simulink model "BuckBoost1"  (Simulink 8.0)
settings: Solver=FixedStepDiscrete  StartTime=0.0  StopTime=5  FixedStep=1e-5  RelTol=1e-3
values from neighbouring files (symbols this model uses):
  Imax = 16    [BuckBoost1_Init1.m]
  R = 30    [BuckBoost1_Init1.m]
  Ts = 1e-3    (= 0.001)    [BuckBoost1_Init1.m]
  Vin = 40    [BuckBoost1_Init1.m]
libraries: powerlib x12, powerlib_extras x2
settings Model: Creator=zxn  LastModifiedBy=Harri
settings DataIOCC: SignalLoggingSaveFormat=ModelDataLogs
settings DebuggingCC: FcnCallInpInsideContextMsg=UseLocalSettings
settings GRTTargetCC: CombineOutputUpdateFcns=off  GRTInterface=on

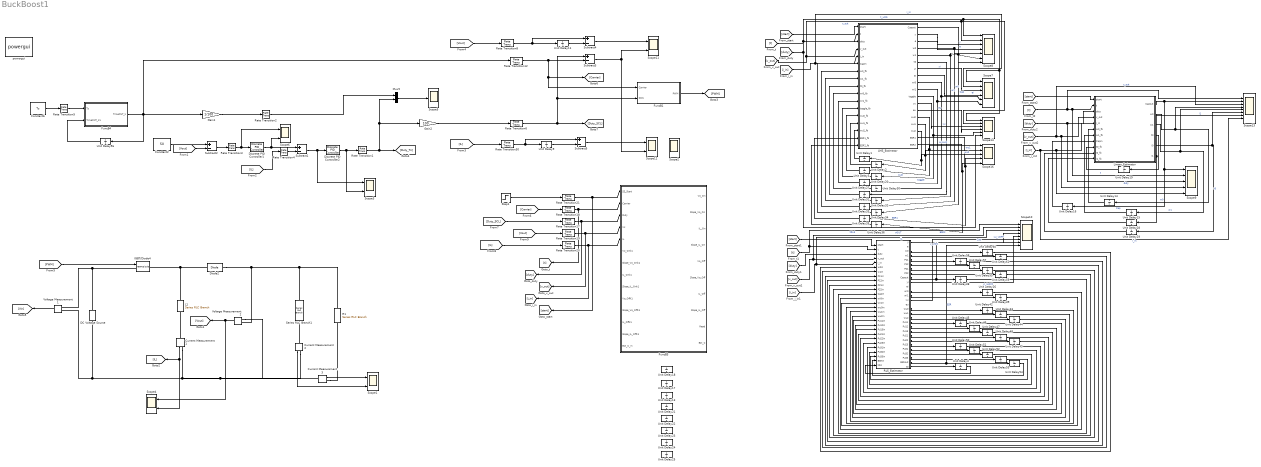
== system BuckBoost1 ==
  Constant2 : Constant  Value=50
  Constant6 : Constant  Value=Ts
  Current Measurement1 : powerlib/Measurements/Current Measurement  PhasorSimulation=off  OutputType=Complex  PSBequivalent=0
  Current Measurement2 : powerlib/Measurements/Current Measurement  PhasorSimulation=off  OutputType=Complex  PSBequivalent=0
  Current Measurement3 : powerlib/Measurements/Current Measurement  PhasorSimulation=off  OutputType=Complex  PSBequivalent=0
  DC Voltage Source : powerlib/Electrical Sources/DC Voltage Source  Amplitude=Vin  Measurements=None
  Diode2 : powerlib/Power Electronics/Diode  Ron=0.001  Lon=0  Vf=0.8  IC=0  UseSnubber=off  Rs=inf  Cs=inf  Measurements=off
  Discrete PID Controller1 : powerlib_extras/Discrete  Control Blocks/Discrete PID Controller  Kp=1.4  Ki=0.4  Kd=0  TcD=0  Par_Limits=[1 -1]*Imax  Init=0  Ts=Ts
  Discrete PID Controller2 : powerlib_extras/Discrete  Control Blocks/Discrete PID Controller  Kp=30e-3  Ki=50e-3  Kd=0  TcD=0  Par_Limits=[1 -1]*0.9  Init=0  Ts=Ts
  FuncB1 : MATLAB Function  TreatAsAtomicUnit=on
  FuncB3 : MATLAB Function  TreatAsAtomicUnit=on
  FuncB4 : MATLAB Function  TreatAsAtomicUnit=on
  Gain1 : Gain  Gain=1/100
  Gain2 : Gain  Gain=100
  IGBT/Diode4 : powerlib/Power Electronics/IGBT//Diode  Ron=1e-3  Rs=1e5  Cs=inf  Measurements=off
  L1 : powerlib/Elements/Series RLC Branch  LConnTagsString=__new0  RConnTagsString=__new0  BranchType=L  Resistance=1  Inductance=5e-3  SetiL0=off  InitialCurrent=0  Capacitance=1e-6  Setx0=off  InitialVoltage=0  Measurements=None
  LMS_Estimator : MATLAB Function  TreatAsAtomicUnit=on
  Linear_Estimator : MATLAB Function  TreatAsAtomicUnit=on
  Mux5 : Mux  Inputs=2
  R1 : powerlib/Elements/Series RLC Branch  LConnTagsString=__new0  RConnTagsString=__new0  BranchType=R  Resistance=R  Inductance=1e-3  SetiL0=off  InitialCurrent=0  Capacitance=1e-6  Setx0=off  InitialVoltage=0  Measurements=None
  RLS_Estimator : MATLAB Function  TreatAsAtomicUnit=on
  Rate Transition{1..2,6,8,12,17..21,30} (11 alike) : RateTransition  OutPortSampleTime=1e-5
  Rate Transition3 : RateTransition  OutPortSampleTime=Ts
  Rate Transition4 : RateTransition  OutPortSampleTime=Ts
  Rate Transition5 : RateTransition  X0=Ts  OutPortSampleTime=1e-5
  Scope{1,3..4,6,11..12} (6 alike) : Scope  NumInputPorts=2
      Scope1 settings: TickLabels=on  TimeRange=10  YMin=210~0  YMax=320~47.5  SaveName=var1
      Scope11 settings: TickLabels=on  TimeRange=5  YMin=-0.06~-40  YMax=0.07~65  SaveName=var10  MaxDataPoints=1000000
      Scope12 settings: TickLabels=on  TimeRange=5  YMin=-0.011~-40  YMax=0.01~65  SaveName=var13  MaxDataPoints=1000000
      Scope3 settings: TickLabels=on  TimeRange=1.5  YMin=0.5~0  YMax=0.605~1  SaveName=var4
      Scope4 settings: TickLabels=on  YMin=0~-1  YMax=52.5~12  SaveName=var
      Scope6 settings: TickLabels=on  TimeRange=1.5  YMin=0.5~0  YMax=0.605~1  SaveName=var2
  Scope10 : Scope  NumInputPorts=8
      settings: TickLabels=on  TimeRange=5  YMin=0~0~0~49.7~0~-5~-5~-5  YMax=100~0.0015~55~50.1~75~5~5~5  SaveName=var9  MaxDataPoints=1000000
  Scope13 : Scope  NumInputPorts=8
      settings: TickLabels=on  TimeRange=5  YMin=0~-1~49.7~49.7~-5~-5~-5~-5  YMax=100~-0.4~50.1~50.1~5~5~5~5  SaveName=var8  MaxDataPoints=1000000
  Scope14 : Scope  NumInputPorts=6
      settings: TickLabels=on  TimeRange=2  YMin=0~-1~49.7~49.7~-1~-5  YMax=100~-0.4~50.1~50.1~2~5  SaveName=var12  MaxDataPoints=1000000
  Scope16 : Scope  NumInputPorts=5
      settings: TickLabels=on  TimeRange=5  YMin=0~-1~49.7~49.7~-5  YMax=100~-0.4~50.1~50.1~5  SaveName=var15  MaxDataPoints=1000000
  Scope2 : Scope  NumInputPorts=4
      settings: TickLabels=on  TimeRange=5  YMin=-0.011~-40~-5~-5  YMax=0.01~65~5~5  SaveName=var3  MaxDataPoints=1000000
  Scope5 : Scope
      settings: TickLabels=on  TimeRange=1.5  YMin=0.5  YMax=0.605  SaveName=var5  MaxDataPoints=100000
  Scope7 : Scope  NumInputPorts=6
      settings: TickLabels=on  TimeRange=5  YMin=0~-1~49.7~49.7~-0.1~-5  YMax=100~-0.4~50.1~50.1~0.1~5  SaveName=var6  MaxDataPoints=1000000
  Scope8 : Scope  NumInputPorts=7
      settings: TickLabels=on  TimeRange=5  YMin=0~-1~49.7~49.7~-0.1~-5~-5  YMax=100~-0.4~50.1~50.1~0.1~5~5  SaveName=var7  MaxDataPoints=1000000
  Scope9 : Scope  NumInputPorts=5
      settings: TickLabels=on  TimeRange=5  YMin=0~-10~-10~0~0  YMax=5~110~110~100~10  SaveName=var11  MaxDataPoints=1000000
  Series RLC Branch1 : powerlib/Elements/Series RLC Branch  LConnTagsString=__new0  RConnTagsString=__new0  BranchType=RC  Resistance=75e-3*1  Inductance=1e-3  SetiL0=off  InitialCurrent=0  Capacitance=1e-3*1.25  Setx0=off  InitialVoltage=500  Measurements=None
  Step1 : Step  Time=3.3  SampleTime=0
  Subtract1 : Sum  Inputs=+-  SampleTime=Ts
  Subtract{2..5} (4 alike) : Sum  Inputs=+-
  Unit Delay{1..4,9,11,13..36,38..39,42..44,46..48,50..52,54..57,60..61} (47 alike) : UnitDelay  SampleTime=1e-5
  Unit Delay{45,49,53,58..59} (5 alike) : UnitDelay  InitialCondition=100  SampleTime=1e-5
  Voltage Measurement1 : powerlib/Measurements/Voltage Measurement  PhasorSimulation=off  OutputType=Complex  PSBequivalent=0
  Voltage Measurement2 : powerlib/Measurements/Voltage Measurement  PhasorSimulation=off  OutputType=Complex  PSBequivalent=0
  powergui : powerlib/powergui  Priority=2  SimulationMode=Discrete  SolverType=Tustin  SampleTime=1e-5  frequency=60  SPID=off  DisableSnubberDevices=off  DisableRonSwitches=off  DisableVfSwitches=off  SwTol=0  Interpol=off  DisplayEquations=off  FunctionMessages=off  frequencyindice=0  Pbase=100e6  ErrMax=1e-4  Iterations=50  UnitsV=kV  UnitsW=MW  echomessages=off  HookPort=off  EnableUseOfTLC=off  x0status=blocks  RestoreLinks=warning  ResistiveCurrentMeasurement=off  Frange=[0:2:500]  Ylog=off  Xlog=off  ShowGrid=off  save=off  variable=ZData  structure=ScopeData  ZoomFFT=on  StartTime=0.0  cycles=1  DisplayStyle=1  fundamental=60  FreqAxis=off  MaxFrequency=8000  frequencyindicesteady=1  RmsSteady=1  display=off  Ts=0  methode=off
  wires:
  Constant2/1 -> Subtract2/1
  Subtract2/1 -> Rate Transition3/1
  Voltage Measurement2/1 -> Scope4/1, [Vout]
  Current Measurement1/1 -> [IL], Scope4/2
  Current Measurement3/1 -> Scope1/1
  Current Measurement2/1 -> Scope1/2
  Rate Transition2/1 -> Mux5/1
  Rate Transition3/1 -> Discrete PID Controller1/1, Scope6/1
  Discrete PID Controller1/1 -> Subtract1/1, Scope6/2
  Subtract1/1 -> Discrete PID Controller2/1, Scope3/1
  Rate Transition4/1 -> Subtract1/2
  [IL] -> Rate Transition4/1
  [Vout] -> Subtract2/2
  Discrete PID Controller2/1 -> Rate Transition1/1, Scope3/2
  Rate Transition1/1 -> Mux5/2, Gain2/1, [Duty_Ts]
  Mux5/1 -> Scope5/1
  Rate Transition6/1 -> [Duty_SCL], Subtract3/1, FuncB1/2(Duty)
  Rate Transition8/1 -> Unit Delay11/1, Subtract4/1
  [PWM] -> IGBT/Diode4/1
  Voltage Measurement1/1 -> [Vin]
  Rate Transition5/1 -> FuncB4/1(Ts)
  Constant6/1 -> Rate Transition5/1
  Unit Delay56/1 -> FuncB4/2(TimeCNT_k1)
  FuncB4/1(TimeCNT_k) -> Unit Delay56/1, Gain1/1, Rate Transition12/1
  Gain1/1 -> Rate Transition2/1
  Gain2/1 -> Rate Transition6/1
  Subtract3/1 -> Scope11/2, Scope12/2
  Rate Transition12/1 -> Subtract3/2, [Carrier], FuncB1/1(Carrier)
  Unit Delay11/1 -> Subtract4/2
  Subtract4/1 -> Scope11/1
  [Vout] -> Rate Transition8/1
  [Carrier] -> Rate Transition18/1
  [Duty_SCL] -> Rate Transition17/1
  Step1/1 -> Rate Transition21/1
  [IL] -> Rate Transition20/1
  [Vout] -> Rate Transition19/1
  FuncB1/1(PWM) -> [PWM]
  Rate Transition21/1 -> [start], FuncB3/1(SS_Start)
  Rate Transition19/1 -> [v_out], FuncB3/4(Vc)
  Rate Transition20/1 -> [i_in], FuncB3/5(IL)
  [IL] -> Rate Transition30/1
  Unit Delay9/1 -> Subtract5/2
  Rate Transition30/1 -> Unit Delay9/1, Subtract5/1
  Subtract5/1 -> Scope12/1
  Rate Transition17/1 -> [duty], FuncB3/3(Duty)
  Rate Transition18/1 -> [t], FuncB3/2(Carrier)
  [start] -> RLS_Estimator/1(start)
  [t] -> RLS_Estimator/2(t), Scope10/1  "tRLS"
  [duty] -> RLS_Estimator/3(duty)
  [v_out] -> Scope10/2, RLS_Estimator/4(v_out)  "vOUT"
  [i_in] -> Scope10/3, RLS_Estimator/5(i_in)  "iL"
  [i_in] -> Scope13/8, Scope9/5, Linear_Estimator/5(i_in)  "i_in"
  [v_out] -> Scope13/3, Scope9/4, Linear_Estimator/4(v_out)  "v_out"
  [duty] -> Scope9/3, Linear_Estimator/3(duty)  "duty"
  [t] -> Scope13/1, Scope9/2, Linear_Estimator/2(t)  "t"
  Linear_Estimator/1(Capout) -> Scope13/2, Unit Delay16/1, Scope9/1  "Cap"
  [start] -> Linear_Estimator/1(start)
  Unit Delay14/1 -> Linear_Estimator/6(w0_fb)
  Unit Delay15/1 -> Linear_Estimator/7(w1_fb)
  Unit Delay16/1 -> Linear_Estimator/8(Capin)
  Linear_Estimator/3(w1) -> Scope13/5, Unit Delay15/1  "w1"
  Linear_Estimator/2(w0) -> Scope13/4, Unit Delay14/1  "w0"
  Linear_Estimator/4(t0) -> Unit Delay19/1
  Unit Delay19/1 -> Linear_Estimator/9(t0_fb)
  Linear_Estimator/6(i1) -> Unit Delay28/1, Scope13/7  "i1"
  Unit Delay28/1 -> Linear_Estimator/11(i1_fb)
  Linear_Estimator/5(i0) -> Scope13/6, Unit Delay29/1  "i0"
  Unit Delay29/1 -> Linear_Estimator/10(i0_fb)
  LMS_Estimator/16(wu2) -> Scope16/3, Unit Delay1/1  "wu2"
  Unit Delay1/1 -> LMS_Estimator/15(wu2_fb)
  LMS_Estimator/15(wu1) -> Unit Delay2/1, Scope16/2  "wu1"
  Unit Delay2/1 -> LMS_Estimator/14(wu1_fb)
  LMS_Estimator/14(wu0) -> Scope16/1, Unit Delay3/1  "wu0"
  Unit Delay3/1 -> LMS_Estimator/13(wu0_fb)
  LMS_Estimator/11(toggle) -> Scope14/5, Unit Delay20/1  "toggle"
  Unit Delay20/1 -> LMS_Estimator/12(toggle_fb)
  LMS_Estimator/10(wi1) -> Scope7/6, Unit Delay27/1  "wi1"
  Unit Delay27/1 -> LMS_Estimator/11(wi1_fb)
  LMS_Estimator/9(wi0) -> Scope7/5, Unit Delay30/1  "wi0"
  Unit Delay30/1 -> LMS_Estimator/10(wi0_fb)
  LMS_Estimator/6(t0) -> Unit Delay31/1
  Unit Delay31/1 -> LMS_Estimator/9(t0_fb)
  LMS_Estimator/5(w1) -> Unit Delay32/1, Scope8/6  "w1"
  Unit Delay32/1 -> LMS_Estimator/8(w1_fb)
  LMS_Estimator/4(w0) -> Scope8/5, Unit Delay33/1  "w0"
  Unit Delay33/1 -> LMS_Estimator/7(w0_fb)
  LMS_Estimator/1(Capout) -> Scope8/7, Unit Delay34/1  "Cap"
  Unit Delay34/1 -> LMS_Estimator/6(Capin)
  [start] -> LMS_Estimator/1(start)
  [t] -> Scope8/1, Scope14/1, Scope7/1, LMS_Estimator/2(t)  "t_LMS"
  [duty] -> Scope14/6, LMS_Estimator/3(duty)
  [v_out] -> Scope14/2, Scope8/2, LMS_Estimator/4(v_out)  "v_out"
  [i_in] -> LMS_Estimator/5(i_in), Scope7/2  "i_in"
  LMS_Estimator/2(y) -> Scope8/3  "y"
  LMS_Estimator/3(e) -> Scope8/4  "e"
  LMS_Estimator/7(yi) -> Scope7/3  "yi"
  LMS_Estimator/8(ei) -> Scope7/4  "ei"
  LMS_Estimator/12(yu) -> Scope14/3  "yu"
  LMS_Estimator/13(eu) -> Scope14/4  "eu"
  LMS_Estimator/17(ESR1) -> Unit Delay35/1, Scope16/4  "ESR1"
  LMS_Estimator/18(ESR2) -> Unit Delay36/1, Scope16/5  "ESR2"
  Unit Delay35/1 -> LMS_Estimator/16(ESR1_fb)
  Unit Delay36/1 -> LMS_Estimator/17(ESR2_fb)
  RLS_Estimator/3(w0) -> Unit Delay60/1
  RLS_Estimator/4(w1) -> Unit Delay61/1
  RLS_Estimator/5(P11) -> Unit Delay58/1
  RLS_Estimator/6(P12) -> Unit Delay57/1
  RLS_Estimator/7(P21) -> Unit Delay55/1
  RLS_Estimator/8(P22) -> Unit Delay59/1
  RLS_Estimator/28(ESRout) -> Scope10/8, Unit Delay54/1  "ESR"
  RLS_Estimator/27(Pu33) -> Unit Delay53/1
  RLS_Estimator/26(Pu32) -> Unit Delay52/1
  RLS_Estimator/25(Pu31) -> Unit Delay51/1
  RLS_Estimator/24(Pu23) -> Unit Delay50/1
  RLS_Estimator/23(Pu22) -> Unit Delay49/1
  RLS_Estimator/22(Pu21) -> Unit Delay48/1
  RLS_Estimator/21(Pu13) -> Unit Delay47/1
  RLS_Estimator/20(Pu12) -> Unit Delay46/1
  RLS_Estimator/19(Pu11) -> Unit Delay45/1
  RLS_Estimator/18(wu2) -> Unit Delay44/1
  RLS_Estimator/17(wu1) -> Unit Delay43/1
  RLS_Estimator/16(wu0) -> Unit Delay42/1
  RLS_Estimator/13(wi1) -> Unit Delay39/1
  RLS_Estimator/12(wi0) -> Unit Delay26/1
  RLS_Estimator/9(Capout) -> Scope10/7, Unit Delay38/1  "Cap"
  Unit Delay54/1 -> RLS_Estimator/27(ESRin)
  Unit Delay53/1 -> RLS_Estimator/26(Pu33in)
  Unit Delay52/1 -> RLS_Estimator/25(Pu32in)
  Unit Delay51/1 -> RLS_Estimator/24(Pu31in)
  Unit Delay50/1 -> RLS_Estimator/23(Pu23in)
  Unit Delay49/1 -> RLS_Estimator/22(Pu22in)
  Unit Delay48/1 -> RLS_Estimator/21(Pu21in)
  Unit Delay47/1 -> RLS_Estimator/20(Pu13in)
  Unit Delay46/1 -> RLS_Estimator/19(Pu12in)
  Unit Delay45/1 -> RLS_Estimator/18(Pu11in)
  Unit Delay44/1 -> RLS_Estimator/17(wu2in)
  Unit Delay43/1 -> RLS_Estimator/16(wu1in)
  Unit Delay42/1 -> RLS_Estimator/15(wu0in)
  Unit Delay39/1 -> RLS_Estimator/14(wi1in)
  Unit Delay26/1 -> RLS_Estimator/13(wi0in)
  Unit Delay38/1 -> RLS_Estimator/12(Capin)
  Unit Delay59/1 -> RLS_Estimator/11(P22in)
  Unit Delay55/1 -> RLS_Estimator/10(P21in)
  Unit Delay57/1 -> RLS_Estimator/9(P12in)
  Unit Delay58/1 -> RLS_Estimator/8(P11in)
  Unit Delay61/1 -> RLS_Estimator/7(w1in)
  Unit Delay60/1 -> RLS_Estimator/6(w0in)
  RLS_Estimator/1(y) -> Scope10/4  "y_vON"
  RLS_Estimator/10(yi) -> Scope10/5  "yi_iLOFF"
  RLS_Estimator/14(yu) -> Scope10/6  "yu_vOFF"
  RLS_Estimator/29(t0) -> Unit Delay4/1
  Unit Delay4/1 -> RLS_Estimator/28(t0in)
  connections:
  DC Voltage Source/RConn1 -- IGBT/Diode4/LConn1 -- Voltage Measurement1/LConn1
  Diode2/RConn1 -- IGBT/Diode4/RConn1 -- L1/RConn1
  Current Measurement3/LConn1 -- Current Measurement2/RConn1 -- Voltage Measurement2/LConn1 -- Current Measurement1/RConn1 -- DC Voltage Source/LConn1 -- Voltage Measurement1/LConn2
  Current Measurement1/LConn1 -- L1/LConn1
  Diode2/LConn1 -- R1/RConn1 -- Series RLC Branch1/RConn1 -- Voltage Measurement2/LConn2
  Current Measurement2/LConn1 -- Series RLC Branch1/LConn1
  Current Measurement3/RConn1 -- R1/LConn1

== matlab function LMS_Estimator ==
  data: start input double; t input double; duty input double; Capout output double; y output double; e output double; v_out input double; i_in input double; Capin input double; w0_fb input double; w1_fb input double; w0 output double; w1 output double; t0_fb input double; t0 output double; yi output double; ei output double; wi0_fb input double; wi1_fb input double; wi0 output double; wi1 output double; toggle_fb input double; wu0_fb input double; wu1_fb input double; wu2_fb input double; toggle output double; yu output double; eu output double; wu0 output double; wu1 output double; wu2 output double; ESR1 output double; ESR2 output double; ESR1_fb input double; ESR2_fb input double
function [Capout, y, e, w0, w1, t0, yi, ei, wi0, wi1, toggle, yu, eu, wu0, wu1, wu2, ESR1, ESR2]  = Est_LMS(start,t,duty,v_out,i_in, Capin, w0_fb, w1_fb, t0_fb, wi0_fb, wi1_fb, toggle_fb, wu0_fb, wu1_fb, wu2_fb, ESR1_fb, ESR2_fb)
%#codegen

% LMS parameter
beta = 0.5;
%(good, let see other value)0.1;
%(good, but w1 still oscilating)0.01;
%(better-but-wrong)0.001;%0.0000001;

% timing control
offset = t - duty;

OFFSET_ON_START_abs = 0+5; % for t
OFFSET_ON_END_rel = -5; % for offset
OFFSET_OFF_START_rel = 5; % for offset
OFFSET_OFF_END_abs = 90+5; % for t


% estimate uoON(t) = w0 + w1*t
y = 0.0;
e = 0.0;
w = transpose(zeros(1,2));
w(1) = w0_fb;
w(2) = w1_fb;
w0 = w0_fb;
w1 = w1_fb;

% estimate iLOFF(t) = wi0 + wi1*t
yi = 0.0;
ei = 0.0;

wi = transpose(zeros(1,2));
wi(1) = wi0_fb;
wi(2) = wi1_fb;
wi0 = wi0_fb;
wi1 = wi1_fb;

% estimate uoOFF(t) = wu0 + wu1*t + wu2*t^2
yu = 0.0;
eu = 0.0;

wu = transpose(zeros(1,3));
wu(1) = wu0_fb;
wu(2) = wu1_fb;
wu(3) = wu2_fb;
wu0 = wu0_fb;
wu1 = wu1_fb;
wu2 = wu2_fb;

% ---

% input for uoON(t) and iLOFF(t), i.e. first-order
x = transpose(zeros(1,2));
x(1) = 1;
x(2) = t;
% input for uoOFF(t), i.e. second-order
u = transpose(zeros(1,3));
u(1) = 1;
u(2) = t;
u(3) = t*t;

% some storage...
t0 = t0_fb;
toggle = toggle_fb;
Capout = Capin; %0; % to avoid error on "unconnected path... something..."

% misc
ESR1 = ESR1_fb;
ESR2 = ESR2_fb;

if(start==1)
    if(toggle == 0)
        % FIRST cycle
        
        if(t > OFFSET_ON_START_abs && offset < OFFSET_ON_END_rel) % ON
            % estimate the "C"
            if (t <= OFFSET_ON_START_abs+2) % give some margin
                t0 = t;
            end
            % --- start of LMS_for_uON(t) ---
            % IMPORTANT: offsetting to zero give good estimation result!
            x(2) = t - t0;

            rms = (x(1)^2+x(2)^2)/2;
            y = w'*x;

            e = v_out - y;

            w = w + beta*e*x/rms;
            w0 = w(1);
            w1 = w(2);
            % --- end of LMS_for_uON(t) ---

        elseif(offset >= OFFSET_ON_END_rel && offset <= OFFSET_ON_END_rel+1)
            Capout = -w0/w1/30*10^(-6) * 1000;%R=30
        end
        if(offset > OFFSET_OFF_START_rel && t < OFFSET_OFF_END_abs) % OFF
            % estimate the "ESR"
            if (offset <= OFFSET_OFF_START_rel+2)
                t0 = t;
            end

            % --- start of LMS_for_iL(t) ---
            x(2) = t - t0;

            rms = (x(1)^2+x(2)^2)/2;
            yi = wi'*x;

            ei = i_in - yi;

            wi = wi + beta*ei*x/rms;
            wi0 = wi(1);
            wi1 = wi(2);
            % --- end of LMS_for_iL(t)---
        %elseif(t >= OFFSET_OFF_END_abs && t <= OFFSET_OFF_END_abs+2)
        %    toggle = 1;
        end
        
        if(t >= OFFSET_OFF_END_abs && t <= OFFSET_OFF_END_abs+2)
            toggle = 1;
        end
        
    elseif(toggle == 1)
        % SECOND cycle
        
        if(offset > OFFSET_OFF_START_rel && t < OFFSET_OFF_END_abs) % OFF
            % estimate the u0(t) in OFF condition
            if (offset <= OFFSET_OFF_START_rel+2)
                t0 = t;
            end

            % --- start of LMS_for_uoOFF(t) ---
            u(2) = t - t0;
            u(3) = (t - t0)*(t - t0);

            rms = (u(1)^2+u(2)^2+u(3)^2)/3;
            yu = wu'*u;

            eu = v_out - yu;

            wu = wu + beta*eu*u/rms;
            wu0 = wu(1);
            wu1 = wu(2);
            wu2 = wu(3);
            % --- end of LMS_for_uoOFF(t)---
        elseif(t >= OFFSET_OFF_END_abs && t <= OFFSET_OFF_END_abs+1)
            %toggle = 0;
            
            R = 30;
            C = Capin;
            a = (2*wu2_fb - wi1_fb*R) / (-wu1_fb - wi1_fb*R*R*C + wi0_fb*R*C*C);
            ESR1 = 1/(a*C) - R;
            
            b = a*wu1_fb + 2*wu2_fb;
            ESR2 = (wi0_fb*C - b) / ((b/R) - wi1_fb);
        end
        
        if(t >= OFFSET_OFF_END_abs && t <= OFFSET_OFF_END_abs+2)
            toggle = 0;
        end
    end
end

== matlab function FuncB3 ==
  data: SS_Start input double; Carrier input double; Duty input double; Vc input double; IL input double; Vo_Onk1 input double; Slope_Vo_Onk1 input double; IL_Onk1 input double; Slope_IL_Onk1 input double; Vo_Offk1 input double; Slope_Vo_Offk1 input double; IL_Offk1 input double; Vo_On output double; Slope_Vo_On output double; IL_On output double; Slope_IL_On output double; Vo_Off output double; Slope_Vo_Off output double; IL_Off output double; Slope_IL_Off output double; Read output double; Slope_IL_Offk1 input double; Est_C output double; Est_C_in input double
function [Vo_On,Slope_Vo_On,IL_On,Slope_IL_On,Vo_Off,Slope_Vo_Off,IL_Off,Slope_IL_Off,Read, Est_C] = Sample(SS_Start,Carrier,Duty,Vc,IL,Vo_Onk1,Slope_Vo_Onk1,IL_Onk1,Slope_IL_Onk1,Vo_Offk1,Slope_Vo_Offk1,IL_Offk1,Slope_IL_Offk1, Est_C_in)

Err1=(Carrier - Duty);  Tsimulation=1e-6;
%DtT_On=Duty*Tsimulation;    DtT_Off=(100 - Duty)*Tsimulation;%%!! 100 should be repaced Correspondingly by CNT_Max
Fix10us=10e-6;
Est_C=Est_C_in;
%Test_Out=Test_Out_in;
if(SS_Start==1)
    if(Err1>=-12)&&(Err1<-11) %%Just After Switch-On; (Err1>=-2)&&(Err1<-1); (Carrier==3)
        Vo_On=Vc; IL_On=IL;
        Read=0;
        Slope_Vo_On=Slope_Vo_Onk1; Slope_IL_On=Slope_IL_Onk1;
        Slope_Vo_Off=Slope_Vo_Offk1; Slope_IL_Off=Slope_IL_Offk1;
        Vo_Off=Vo_Offk1; IL_Off=IL_Offk1;
        Est_C=1;
    elseif((Err1>=-2)&&(Err1<-1)) %%Next moment Switch-Off
        %Slope_Vo_On=(Vc - Vo_Onk1)/DtT_On; Slope_IL_On=(IL - IL_Onk1)/DtT_On;
        Slope_Vo_On=(Vc - Vo_Onk1)/Fix10us; Slope_IL_On=(IL - IL_Onk1)/Fix10us;
        Vo_On=Vo_Onk1; IL_On=IL_Onk1;
        Slope_Vo_Off=Slope_Vo_Offk1; Slope_IL_Off=Slope_IL_Offk1; Read=0; 
        Vo_Off=Vo_Offk1; IL_Off=IL_Offk1;
        Est_C=2;
    elseif(Carrier==89) %%Just After Switch Off; Carrier==98; (Err1>3)&&(Err1<=4)
        Vo_Off=Vc;  IL_Off=IL;
        Slope_Vo_Off=Slope_Vo_Offk1;  Slope_IL_Off=Slope_IL_Offk1;
        Slope_Vo_On=Slope_Vo_Onk1;  Slope_IL_On=Slope_IL_Onk1; Read=0;
        Vo_On=Vo_Onk1; IL_On=IL_Onk1;
    elseif(Carrier==99) %%Next moment Switch-On
        %Slope_Vo_Off=(Vc - Vo_Offk1)/DtT_Off;  Slope_IL_Off=(IL - IL_Offk1)/DtT_Off;
        Slope_Vo_Off=(Vc - Vo_Offk1)/Fix10us;  Slope_IL_Off=(IL - IL_Offk1)/Fix10us;
        Vo_Off=Vo_Offk1;  IL_Off=IL_Offk1;
        Read=1;
        Slope_Vo_On=Slope_Vo_Onk1; Slope_IL_On=Slope_IL_Onk1;
        Vo_On=Vo_Onk1; IL_On=IL_Onk1;
    %elseif(Est_C==1)
    %    Test_Out = 2;
    %elseif(Est_C==2)
    %    Test_Out = 3;
    else
        Vo_On=Vo_Onk1; Slope_Vo_On=Slope_Vo_Onk1; IL_On=IL_Onk1; Slope_IL_On=Slope_IL_Onk1; %%On_Readk1
        Vo_Off=Vo_Offk1;  Slope_Vo_Off=Slope_Vo_Offk1;  IL_Off=IL_Offk1;  Slope_IL_Off=Slope_IL_Offk1; Read=0; %%Off_Readk1
    end
else
    Vo_On=49;  Slope_Vo_On=0.5;  IL_On=4;  Slope_IL_On=0.2;
    Vo_Off=50;  Slope_Vo_Off=0.5;  IL_Off=3.8;  Slope_IL_Off=0.2; Read=0;
end

end

== matlab function RLS_Estimator ==
  data: y output double; e output double; w0 output double; w1 output double; P11 output double; P12 output double; P21 output double; P22 output double; Capout output double; start input double; t input double; duty input double; v_out input double; i_in input double; w0in input double; w1in input double; P11in input double; P12in input double; P21in input double; P22in input double; Capin input double; wi0in input double; wi1in input double; wu0in input double; wu1in input double; wu2in input double; Pu11in input double; Pu12in input double; Pu13in input double; Pu21in input double; Pu22in input double; Pu23in input double; Pu31in input double; Pu32in input double; Pu33in input double; ESRin input double; yi output double; ei output double; wi0 output double; wi1 output double; yu output double; eu output double; wu0 output double; wu1 output double; wu2 output double; Pu11 output double; Pu12 output double; Pu13 output double; Pu21 output double; Pu22 output double; Pu23 output double; Pu31 output double; Pu32 output double; Pu33 output double; ESRout output double; t0in input double; t0 output double
function [y, e, w0, w1, P11, P12, P21, P22, Capout, yi, ei, wi0, wi1, yu, eu, wu0, wu1, wu2, Pu11, Pu12, Pu13, Pu21, Pu22, Pu23, Pu31, Pu32, Pu33, ESRout, t0]  = Est_RLS(start,t,duty,v_out,i_in, w0in, w1in, P11in, P12in, P21in, P22in, Capin, wi0in, wi1in, wu0in, wu1in, wu2in, Pu11in, Pu12in, Pu13in, Pu21in, Pu22in, Pu23in, Pu31in, Pu32in, Pu33in, ESRin, t0in)
%#codegen

% --- Time Partition ---
sampling_time = 1e-5;% 1e-6;

offset = t - duty;

OFFSET_ON_START_abs = 0+5; % for t
OFFSET_ON_END_rel = -5; % for offset
OFFSET_OFF_START_rel = 5; % for offset
OFFSET_OFF_END_abs = 90+5; % for t
% --- end of Time Partition ---

% --- Init ---
lambda = 0.6;
% good for change: 0.7; not good with change: 0.999;
delta = 1/100;

% <<--- uON(t) = w0 + w1*t --->>

% ... estimator output ...
y = 0.0;
e = 0.0;

% ... inputs ...
u = transpose(zeros(1,2));
u(1) = 1;
u(2) = t;

% ... coefficients ...
w = zeros(2,1);
w(1) = w0in;
w(2) = w1in;
w0 = w0in; w1 = w1in;

% ... algorithm specific tools ...
P = eye(2) / delta;
P(1,1) = P11in; P(1,2) = P12in;
P(2,1) = P21in; P(2,2) = P22in;
%NOTE: in "delay unit" blocks, set:
% P11in and P22in --> 100 (as per 'delta')
% P12in and P21in --> 0 (since "eye" matrix)
P11 = P11in; P12 = P12in;
P21 = P21in; P22 = P22in;

% <<--- iLOFF(t) = wi0 + wi1*t --->>

% ... estimator output ...
yi = 0.0;
ei = 0.0;

% ... inputs ...
% REUSE

% ... coefficients ...
wi = zeros(2,1);
wi(1) = wi0in;
wi(2) = wi1in;
wi0 = wi0in; wi1 = wi1in;

% ... algorithm specific tools ...
% REUSE

% <<--- uON(t) = wu0 + wu1*t + wu2*t^2 --->>

% ... estimator output ...
yu = 0.0;
eu = 0.0;

% ... inputs ...
uu = transpose(zeros(1,3));
uu(1) = 1;
uu(2) = t;
uu(3) = t*t;

% ... coefficients ...
wu = zeros(3,1);
wu(1) = wu0in;
wu(2) = wu1in;
wu(3) = wu2in;
wu0 = wu0in; wu1 = wu1in; wu2 = wu2in;

% ... algorithm specific tools ...
Pu = eye(3) / delta;
% TODO: remove P(i,j) with i!=j...
Pu(1,1) = Pu11in; Pu(1,2) = Pu12in; Pu(1,3) = Pu13in;
Pu(2,1) = Pu21in; Pu(2,2) = Pu22in; Pu(2,3) = Pu23in;
Pu(3,1) = Pu31in; Pu(3,2) = Pu32in; Pu(3,3) = Pu33in;
%NOTE: in "delay unit" blocks, set:
% P11in and P22in --> 100 (as per 'delta')
% P12in and P21in --> 0 (since "eye" matrix)
Pu11 = Pu11in; Pu12 = Pu12in; Pu13 = Pu13in;
Pu21 = Pu21in; Pu22 = Pu22in; Pu23 = Pu23in;
Pu31 = Pu31in; Pu32 = Pu32in; Pu33 = Pu33in;

% --- end of Init ---

% --- Feedback ---

Capout = Capin;
ESRout = ESRin;
t0 = t0in;
% --- end of Feedback ---

noiseAmp = 0; % rand : [0,1]

if(start==1)
    if(t > OFFSET_ON_START_abs && offset < OFFSET_ON_END_rel) % ON
        % estimate the "C"
        if(t > OFFSET_ON_START_abs && t<= OFFSET_ON_START_abs+2)
            t0 = t;
        else
            % --- start of RLS for uON(t) ---
            %u(2) = t - t0; NOTE: RLS do not require this kind of offsetting!
            u(2) = (t - t0) * sampling_time; %NOTE: not necessary to offset!
            k = ( (P*u) / (1 + (u' * P * u) / lambda) ) / lambda;
            y = w' * u;
            %e = v_out - y;
            e = (v_out + (noiseAmp*rand)) - y;

            w = w + k*e;
            w0 = w(1); w1 = w(2);

            P = ( P - k * u' * P ) / lambda;
            P11 = P(1,1); P12 = P(1,2);
            P21 = P(2,1); P22 = P(2,2);
            % --- end of RLS for uON(t) ---
        end
    end
    if(offset >= OFFSET_ON_END_rel && offset <= OFFSET_ON_END_rel+1)
        Capout = -w0/w1/30;%*sampling_time;%R=30
    end
    
    if(offset > OFFSET_OFF_START_rel && t < OFFSET_OFF_END_abs) % OFF
        % estimate the "ESR"
        if(offset > OFFSET_OFF_START_rel && offset <= OFFSET_OFF_START_rel+2)
            t0 = t;
        else
            % --- start RLS for iLOFF(t) ---
            u(2) = (t - t0) * sampling_time; %NOTE: not necessary to offset!
            k = ( (P*u) / (1 + (u' * P * u) / lambda) ) / lambda;
            yi = wi' * u;
            %ei = i_in - yi;
            ei = (i_in + (noiseAmp*rand)) - yi;

            wi = wi + k*ei;
            wi0 = wi(1); wi1 = wi(2);

            P = ( P - k * u' * P ) / lambda;
            P11 = P(1,1); P12 = P(1,2);
            P21 = P(2,1); P22 = P(2,2);
            % --- end of RLS for iLOFF(t) ---

            % --- start RLS for uOFF(t) ---
            uu(2) = (t - t0) * sampling_time; %NOTE: not necessary to offset!
            uu(3) = uu(2)*uu(2);
            ku = ( (Pu*uu) / (1 + (uu' * Pu * uu) / lambda) ) / lambda;
            yu = wu' * uu;
            %eu = v_out - yu;
            eu = (v_out + (noiseAmp*rand)) - yu;

            wu = wu + ku*eu;
            wu0 = wu(1); wu1 = wu(2); wu2 = wu(3);

            Pu = ( Pu - ku * uu' * Pu ) / lambda;
            Pu11 = Pu(1,1); Pu12 = Pu(1,2); Pu13 = Pu(1,3);
            Pu21 = Pu(2,1); Pu22 = Pu(2,2); Pu23 = Pu(2,3);
            Pu31 = Pu(3,1); Pu32 = Pu(3,2); Pu33 = Pu(3,3);
            % --- end of RLS for uOFF(t) ---
        end
    end
    if(t >= OFFSET_OFF_END_abs && t <= OFFSET_OFF_END_abs+1)
        a = 2*wu2 / (wi1*30 - wu1);
        b = 2*wu2 / (1 - wu1/30/wi1);
        c = wu0*a + b/a - 2*wu2/a;
        ESRout = (wi0/Capin - c) / (c/30 - wi1);
    end

end

== matlab function Linear_Estimator ==
  data: start input double; t input double; duty input double; Capout output double; v_out input double; i_in input double; w0_fb input double; w1_fb input double; w0 output double; w1 output double; Capin input double; t0_fb input double; t0 output double; i0_fb input double; i1_fb input double; i0 output double; i1 output double
function [Capout, w0, w1, t0, i0, i1]  = Est_Linear(start,t,duty,v_out,i_in, w0_fb, w1_fb, Capin, t0_fb, i0_fb, i1_fb)
%#codegen

%beta = 0.5;
%(good, let see other value)0.1;
%(good, but w1 still oscilating)0.01;
%(better-but-wrong)0.001;%0.0000001;

offset = t - duty;

OFFSET_ON_START_abs = 0+5; % for t
OFFSET_ON_END_rel = -5; % for offset
OFFSET_OFF_START_rel = 5; % for offset
OFFSET_OFF_END_abs = 90+5; % for t

Capout = Capin; %0; % to avoid error on "unconnected path... something..."

w0 = w0_fb;
w1 = w1_fb;
t0 = t0_fb;
i0 = i0_fb;
i1 = i1_fb;

if(start==1)
    if(t > OFFSET_ON_START_abs && offset < OFFSET_ON_END_rel) % ON
        % estimate the "C"
        if (t <= OFFSET_ON_START_abs+2) % give some margin
            t0 = t;
            w0 = v_out;
        end
    elseif(offset >= OFFSET_ON_END_rel-1 && offset <= OFFSET_ON_END_rel+1)
        w1 = (v_out - w0)/(t - t0);
        Capout = -w0/w1/30*10^(-6) * 1000;%R=30
        
    elseif(offset > OFFSET_OFF_START_rel && t < OFFSET_OFF_END_abs) %OFF
        if (offset <= OFFSET_OFF_START_rel+2)
            t0 = t;
            i0 = i_in;
        end
    elseif(t >= OFFSET_OFF_END_abs-1 && t <= OFFSET_OFF_END_abs)
        i1 = (i_in - i0)/(t - t0);
    end
else
    % initiate the coefficients
end

== matlab function FuncB1 ==
  data: PWM output double; Carrier input double; Duty input double
function PWM  = Sample(Carrier,Duty)

Err1=(Duty - Carrier);
%%Single Switch PWM Signal Generation!
if(Err1>0)
    PWM=1;
else
    PWM=0;
end

end

== matlab function FuncB4 ==
  data: Ts input double; TimeCNT_k1 input double; TimeCNT_k output double
function TimeCNT_k  = IabSlope(Ts,TimeCNT_k1)

Tsimulation=1e-5;%1e-6;
CNT_Ts=Ts/Tsimulation - 1; %%100
%%Vap,Vbt Calculation
if(TimeCNT_k1>=CNT_Ts)
    TimeCNT_k=0;
else
    TimeCNT_k=TimeCNT_k1 + 1;
end

end
